simulink model "dc_motor_kalman_filter_validation"  (R2021a)
settings: Solver=VariableStepAuto  StartTime=0.0  StopTime=40.0  RelTol=1e-3
values from neighbouring files (symbols this model uses):
  R_kf = eye(2)    [dc_motor_control.m]    (also in rotating_pendulum_3states.m = 10 * diag([1, 1, 10]); rotating_pendulum_4states.m = diag([7.5740e-06, 0.1526, 1.4489e-05, 0.2930]))
  theta1 = conv_theta(theta1)    [dc_motor_control.m]    (also in identification_dc_motor.m; model_identification_dcmotor.m; model_identification_simplified.m; visualize_data.m)
undefined symbols (not defined in the file or in its folder): Discrete, Time
libraries: ctrlSharedLib x1
settings Model: Creator=danny  LastModifiedBy=danny

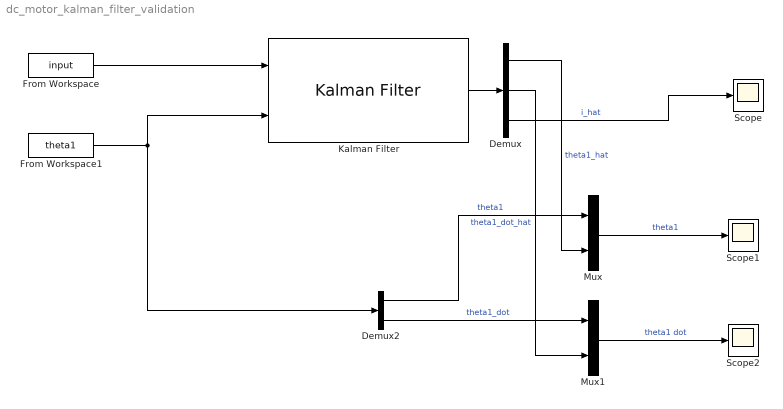
== system dc_motor_kalman_filter_validation ==
  Demux : Demux  Outputs=3
  Demux2 : Demux  Outputs=2
  From Workspace : FromWorkspace  VariableName=input  SampleTime=0.001
  From Workspace1 : FromWorkspace  VariableName=theta1  SampleTime=0.001
  Kalman Filter : ctrlSharedLib/Kalman Filter  TimeDomain=Discrete-Time  UseCurrentEstimator=on  ModelSource=LTI State-Space Variable  ModelSourceVariable=dc_motor_ss  A=0.95  B=1  C=1  D=0  NumberOfStates=1  NumberOfInputs=1  NumberOfOutputs=1  InitialEstimateSource=Dialog  X0=[theta1.Data(1,1), theta1.Data(2,1), 0.0]  P0=10  UseK=off  UseGH=off  NumberOfProcessNoiseInputs=1  G=1  TimeInvariantG=on  H=0  TimeInvariantH=on  Q=Q_kf  TimeInvariantQ=on  R=R_kf  TimeInvariantR=on  N=0  TimeInvariantN=on  AddInputPort=on  AddEnablePort=off  OutputEstimatedY=off  OutputP=off  Ts=-1
  Mux : Mux  Inputs=2
  Mux1 : Mux  Inputs=2
  Scope : Scope
  Scope1 : Scope
  Scope2 : Scope
  wires:
  From Workspace/1 -> Kalman Filter/1
  Mux/1 -> Scope1/1  "theta1"
  Mux1/1 -> Scope2/1  "theta1 dot"
  From Workspace1/1 -> Demux2/1, Kalman Filter/2
  Kalman Filter/1 -> Demux/1
  Demux/3 -> Scope/1  "i_hat"
  Demux/1 -> Mux/2  "theta1_hat"
  Demux2/1 -> Mux/1  "theta1"
  Demux2/2 -> Mux1/1  "theta1_dot"
  Demux/2 -> Mux1/2  "theta1_dot_hat"
